simulink model "sirmodel"  (Simulink 7.9)
settings: Solver=ode45  StartTime=0.0  StopTime=10.0  RelTol=1e-6
values from neighbouring files (symbols this model uses):
  b = 0.2    [predprey.m]    (also in sir.m = 0.003)
  I0 = 50    [sir.m]
  r = 10    [lim_grow_script.m]    (also in sir.m = 0.55)
  R0 = 0    [sir.m]
  S0 = 1450    [sir.m]
settings Model: Creator=Daniel  LastModifiedBy=Daniel

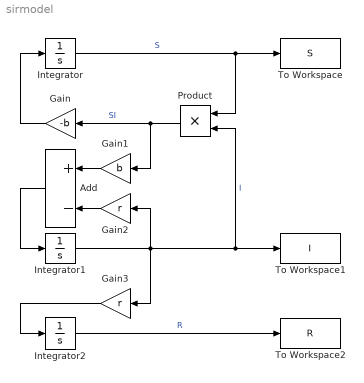
== system sirmodel ==
  Add : Sum  Inputs=+-
  Gain : Gain  Gain=-b
  Gain1 : Gain  Gain=b
  Gain2 : Gain  Gain=r
  Gain3 : Gain  Gain=r
  Integrator : Integrator  InitialCondition=S0
  Integrator1 : Integrator  InitialCondition=I0
  Integrator2 : Integrator  InitialCondition=R0
  Product : Product  RndMeth=Zero
  To Workspace : ToWorkspace  VariableName=S  SampleTime=-1
  To Workspace1 : ToWorkspace  VariableName=I  SampleTime=-1
  To Workspace2 : ToWorkspace  VariableName=R  SampleTime=-1
  wires:
  Gain/1 -> Integrator/1
  Integrator/1 -> Product/1, To Workspace/1  "S"
  Integrator1/1 -> Gain2/1, Gain3/1, Product/2, To Workspace1/1  "I"
  Product/1 -> Gain/1, Gain1/1  "SI"
  Gain1/1 -> Add/1
  Gain2/1 -> Add/2
  Add/1 -> Integrator1/1
  Gain3/1 -> Integrator2/1
  Integrator2/1 -> To Workspace2/1  "R"
